simulink model "PSKDemodulator"  (R2024a)
settings: Solver=VariableStepAuto  StartTime=0.0  StopTime=10.0  RelTol=1e-3
settings Model: Creator=prath  LastModifiedBy=prath

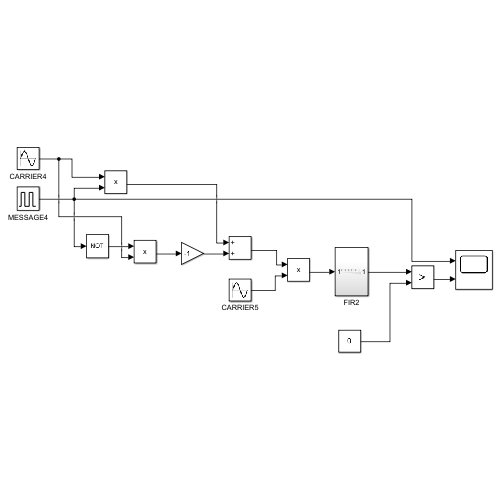
[thumbnail: Simulink's stored preview of the top-level diagram]
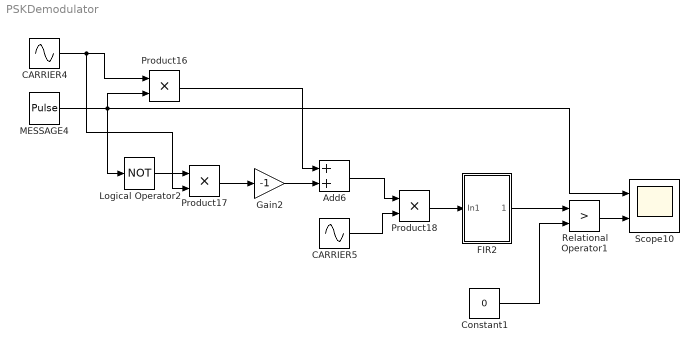
== system PSKDemodulator ==
  Add6 : Sum
  CARRIER4 : Sin  Frequency=100  SampleTime=0
  CARRIER5 : Sin  Frequency=100  SampleTime=0
  Constant1 : Constant  Value=0
  FIR2 : Subsystem
  Gain2 : Gain  Gain=-1
  Logical Operator2 : Logic  Operator=NOT  AllPortsSameDT=off  OutDataTypeStr=boolean
  MESSAGE4 : DiscretePulseGenerator  PulseType=Time based  Period=1  PulseWidth=50
  Product16 : Product
  Product17 : Product
  Product18 : Product
  Relational Operator1 : RelationalOperator  Operator=>  OutDataTypeStr=boolean  RndMeth=Simplest  InputSameDT=off
  Scope10 : Scope  NumInputPorts=2
  wires:
  Product18/1 -> FIR2/1(In1)
  FIR2/1(Out1) -> Relational Operator1/1
  Product16/1 -> Add6/1
  CARRIER4/1 -> Product17/2, Product16/1
  Logical Operator2/1 -> Product17/1
  Relational Operator1/1 -> Scope10/2
  CARRIER5/1 -> Product18/2
  Add6/1 -> Product18/1
  Product17/1 -> Gain2/1
  MESSAGE4/1 -> Scope10/1, Logical Operator2/1, Product16/2
  Gain2/1 -> Add6/2
  Constant1/1 -> Relational Operator1/2

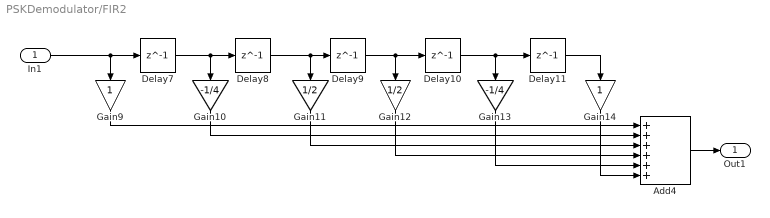
== system PSKDemodulator/FIR2 ==
  In1 : Inport
  Add4 : Sum  Inputs=++++++
  Delay{7..11} (5 alike) : Delay  DelayLength=1
  Gain10 : Gain  Gain=-1/4
  Gain11 : Gain  Gain=1/2
  Gain12 : Gain  Gain=1/2
  Gain13 : Gain  Gain=-1/4
  Gain14 : Gain
  Gain9 : Gain
  Out1 : Outport
  wires:
  Delay8/1 -> Delay9/1, Gain11/1
  Delay10/1 -> Delay11/1, Gain13/1
  Gain10/1 -> Add4/2
  In1/1 -> Gain9/1, Delay7/1
  Gain14/1 -> Add4/6
  Gain13/1 -> Add4/5
  Gain11/1 -> Add4/3
  Gain9/1 -> Add4/1
  Gain12/1 -> Add4/4
  Delay7/1 -> Gain10/1, Delay8/1
  Delay9/1 -> Delay10/1, Gain12/1
  Delay11/1 -> Gain14/1
  Add4/1 -> Out1/1
